simulink model "P90e"  (R2015b)
settings: Solver=VariableStepAuto  StartTime=0.0  StopTime=3  RelTol=1e-3
settings Model: Creator=xmax1946  LastModifiedBy=xmax1946

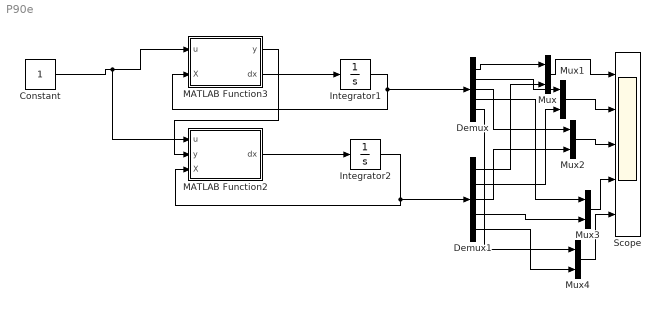
== system P90e ==
  Constant : Constant
  Demux : Demux  Outputs=5
  Demux1 : Demux  Outputs=5
  Integrator1 : Integrator  InitialCondition=[0;0;0;0;0]  IgnoreLimit=on
  Integrator2 : Integrator  InitialCondition=[1;1;1;1;1]
  MATLAB Function2 : MATLAB Function  TreatAsAtomicUnit=on
  MATLAB Function3 : MATLAB Function  TreatAsAtomicUnit=on
  Mux{,1..4} (5 alike) : Mux  Inputs=2
  Scope : Scope  NumInputPorts=5
  wires:
  Constant/1 -> MATLAB Function2/1(u), MATLAB Function3/1(u)
  MATLAB Function2/1(dx) -> Integrator2/1
  MATLAB Function3/2(dx) -> Integrator1/1
  Integrator1/1 -> MATLAB Function3/2(X), Demux/1
  Integrator2/1 -> Demux1/1, MATLAB Function2/3(X)
  MATLAB Function3/1(y) -> MATLAB Function2/2(y)
  Demux/1 -> Mux/1
  Demux1/1 -> Mux/2
  Mux/1 -> Scope/1
  Mux3/1 -> Scope/4
  Demux1/4 -> Mux3/2
  Demux/4 -> Mux3/1
  Mux2/1 -> Scope/3
  Demux1/3 -> Mux2/2
  Demux/3 -> Mux2/1
  Demux/2 -> Mux1/1
  Demux1/2 -> Mux1/2
  Mux1/1 -> Scope/2
  Mux4/1 -> Scope/5
  Demux/5 -> Mux4/1
  Demux1/5 -> Mux4/2

== matlab function P90e/MATLAB Function2 ==
  data: u input; y input; X input; dx output
function dx  = fcn(u,y,X)
A=[0,-1,0,0,-4;0,0,1,0,1;0,1,0,0,2;-2,1,0,-2,4;0,0,0,0,-2];
B=[0;1;0;0;0];
C=[1,0,0,0,0];
L =[10.0000;36.0000;64.0000;48.0000;0];

dx=A*X+B*u+(L*(y-C*X));

== matlab function P90e/MATLAB Function3 ==
  data: u input; y output; X input; dx output
function [y,dx] = fcn(u,X)
A=[0,-1,0,0,-4;0,0,1,0,1;0,1,0,0,2;-2,1,0,-2,4;0,0,0,0,-2];
B=[0;1;0;0;0];
C=[1,0,0,0,0];

dx=A*X+B*u;
y=C*X;
